simulink model "demo5_1"  (R2018b)
settings: Solver=FixedStepAuto  StartTime=0.0  StopTime=10.0  FixedStep=0.01  RelTol=1e-3
settings Model: Creator=Gavin  LastModifiedBy=Gavin
settings OptimizationCC: DefaultParameterBehavior=Inlined  EnhancedBackFolding=on  PassReuseOutputArgsAs=Individual arguments  OptimizeBlockOrder=speed  DifferentSizesBufferReuse=on  OptimizationCustomize=off
settings DebuggingCC: ParameterTunabilityLossMsg=error
settings SFSimCC: MATLABDynamicMemAlloc=off
settings RTWCC: SystemTargetFile=ert.tlc  TemplateMakefile=ert_default_tmf  GenerateReport=on  IncludeHyperlinkInReport=on  LaunchReport=on  GenerateTraceInfo=on  GenerateTraceReport=on  GenerateTraceReportSl=on  GenerateTraceReportSf=on  GenerateTraceReportEml=on
settings CodeAppCC: ForceParamTrailComments=on  IgnoreCustomStorageClasses=off  OperatorAnnotations=on  SimulinkDataObjDesc=on  SFDataObjDesc=on  InsertBlockDesc=on
settings ERTTargetCC: TargetLangStandard=C99 (ISO)  GenerateSampleERTMain=on  InlinedParameterPlacement=NonHierarchical  ERTCustomFileTemplate=example_file_process.tlc

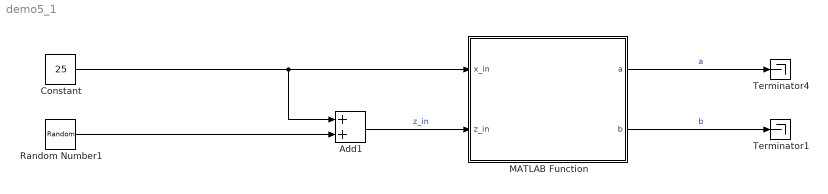
== system demo5_1 ==
  Add1 : Sum
  Constant : Constant  Value=25
  MATLAB Function : MATLAB Function  TreatAsAtomicUnit=on
  Random Number1 : RandomNumber  Variance=0.04  SampleTime=0.01
  Terminator1 : Terminator
  Terminator4 : Terminator
  wires:
  Random Number1/1 -> Add1/2
  MATLAB Function/1(a) -> Terminator4/1  "a"
  Add1/1 -> MATLAB Function/2(z_in)  "z_in"
  Constant/1 -> Add1/1, MATLAB Function/1(x_in)
  MATLAB Function/2(b) -> Terminator1/1  "b"

== matlab function demo5_1/MATLAB Function ==
  data: x_in input; a output; z_in input; b output
function [a,b] = RLS_linear2(x_in,z_in)
% 2 Dim Vector RLS
% By Du QingYa
persistent x P
if isempty(x)
    x = cast([x_in;0],class(z_in));  % state variables initial
    P = cast(0.04*eye(2),class(z_in)); % covariance matrix
end
    H = [1 0.01];
    Z = z_in;
    
    K = P*H'/(H*P*H'+1);
    P = (0.04*eye(2) - K*H)*P;           % covariance matrix P update
    x = x+K*(Z-H*x);               % x state update
    
    a = x(1);
    b = x(2);
end
